simulink model "flightSimulation"  (R2018a)
settings: Solver=FixedStepAuto  StartTime=0  StopTime=end_time  FixedStep=0.005  RelTol=1e-3  EnableMultiTasking=on
values from neighbouring files (symbols this model uses):
  initPosLLA = [37.6287386167 -122.393391133 100]    [cmdh.mat]    (also in cmdyaw.mat)
  mass = 1.53    [cmdh.mat]    (also in cmdyaw.mat)
  Ts = 0.01    [cmdh.mat]    (also in cmdyaw.mat)
undefined symbols (not defined in the file or in its folder): B, Earth, ft, m, p_limits, s, sigbuilder_block, sw_turb, umax, umin, Vehicle, WGS84
libraries: simulink x23, aerolibactuator x15, dspswit3 x12, dspsrcs4 x10, dsparch4 x7, aerolibconvert2 x4, aerolibanimutils x2, qcatlib x2, aerolibfltsims x2, aerolibutil x2, shared6dof x1, aerolibtransform2 x1
(part 4 of 4)

== matlab function flightSimulation/Subsystem/ADRC_allocator1/MATLAB Function ==
  data: x1_d input; u_r output; x2_d input; x1 input; x2 input
function u_r = NLSEF_yaw(x1_d,x2_d,x1,x2)
e1=x1_d-x1;
if e1<-pi
    a1=e1+2*pi;
elseif e1>=pi
    a1=e1-2*pi;
else   
    a1=e1;
end
e2=x2_d-x2;
% kp=0.5;kd=0.5;% 限11
% kp=1;kd=1; % 限20
kp=0.5;kd=0.5;% 噪声
alfa1=0.75;alfa2=1.5;
delta=0.1;
u_r = kp*fal(a1,alfa1,delta)+kd*fal(e2,alfa2,delta); 
% kp=0.5;kd=0.5;
% u_r = kp*a1+kd*e2;   % 控制输出
end

== matlab function flightSimulation/Subsystem/ADRC_allocator1/MATLAB Function2 ==
  data: x1_d input; u_q output; x2_d input; x1 input; x2 input
function u_q = NLSEF_pitch(x1_d,x2_d,x1,x2)
e1=x1_d-x1;
e2=x2_d-x2;
% kp=1;kd=1.5;% 限11
% kp=1.5;kd=2;% 限20
kp=1;kd=1;% 噪声
alfa1=0.75;alfa2=1.5;
delta=0.1;
u_q = kp*fal(e1,alfa1,delta)+kd*fal(e2,alfa2,delta);   % 控制输出
% kp=0.4;kd=0.4;
% u_q = kp*e1+kd*e2;   % 控制输出
end

== matlab function flightSimulation/Subsystem/ADRC_allocator1/MATLAB Function3 ==
  data: x1_d input; u_p output; x2_d input; x1 input; x2 input
function u_p = NLSEF_roll(x1_d,x2_d,x1,x2)
e1=x1_d-x1;
e2=x2_d-x2;
% kp=1;kd=1.5;% 限11
% kp=1.5;kd=2;% 限20
kp=1;kd=1;% 噪声
alfa1=0.75;alfa2=1.5;
delta=0.1;
u_p = kp*fal(e1,alfa1,delta)+kd*fal(e2,alfa2,delta);   % 控制输出
% kp=0.4;kd=0.4;
% u_p = kp*e1+kd*e2;   % 控制输出
end

== matlab function flightSimulation/Subsystem/PID_allocator1/舵机偏角输入eso/MATLAB Function2 ==
  data: u input; y output
function y = fcn(u)
U1=u(1);
U2=u(2);
U3=u(3);
A=0.3491;

D=[-1  0  1;
    0 -1  1;
    1  0  1;
    0  1  1];
% D
D_=1*[-0.5000         0              0.5000         0;
         0           -0.5000         0              0.5000;
       0.2500         0.2500         0.2500         0.2500];
% pinv(D)
kc1=2.7;% 2.8
kc2=3.2;% 3.3
l_1=0.17078793;
l_2=0.06647954;
K=1*[-kc1*l_1    0        kc1*l_1     0;
      0      -kc1*l_1     0        kc1*l_1;
      kc2*l_2   kc2*l_2    kc2*l_2    kc2*l_2];
K_=pinv(K);
I_x=0.025483;
I_y=0.025504;
I_z=0.00562;
I=[I_x 0 0;0 I_y 0;0 0 I_z];
a=A-abs(U1);
b=A-abs(U2);
D_s=[-1  0 (2*a)/(a+b);
      0 -1  (2*b)/(a+b);
      1  0  (2*a)/(a+b);
      0  1 (2*b)/(a+b)];
    D=[-1  0  1;
      0 -1  1;
      1  0  1;
      0  1  1];
y=zeros(3,1);
y=I\(K*D)*([U1;U2;U3]);% K*D=K*D_s
% I\(K*D)*([U1;U2;U3])=扰动角加速度

== matlab function flightSimulation/Subsystem/ADRC_allocator1/Subsystem2/control allocation/inv/inv ==
  data: u input; y output
function y = fcn(u)
U = [u(1);u(2);u(3)];
y=zeros(4,1);
% M=crossover_point([0;0;0],e);
% if (norm(e)>norm(M))
%     U=M;
% else
%     U=e;
% end 
% B=[-0.5   0       0.5   0;
%     0  -0.5    0       0.5;
%     0.25   0.25   0.25   0.25];
kc1=3.157;% 2.8
kc2=3.157;% 3.3
l_1=0.17078793;
l_2=0.06647954;
B=1*[-kc1*l_1    0        kc1*l_1     0;
      0      -kc1*l_1     0        kc1*l_1;
      kc2*l_2   kc2*l_2    kc2*l_2    kc2*l_2];  
% u(1)=Constrain(u(1),umin(1),umax(1));
% u(2)=Constrain(u(2),umin(2),umax(2));
% u(3)=Constrain(u(3),umin(3),umax(3));
% u(4)=Constrain(u(4),umin(4),umax(4));
c=pinv(B)*U;
y=[c(1);c(2);c(3);c(4)];

== matlab function flightSimulation/Subsystem/PID/MATLAB Function ==
  data: u input; y output
function y = Eulerrate2pqr(u)
Roll=u(4);
Pitch=u(5);
Q=[1    sin(Roll)*tan(Pitch)    cos(Roll)*tan(Pitch);
   0        cos(Roll)               -sin(Roll);
   0    sin(Roll)*sec(Pitch)    cos(Roll)*sec(Pitch)];
y = Q\[u(1);u(2);u(3)];

== matlab function flightSimulation/Subsystem/PID/MATLAB Function1 ==
  data: u input; y output
function y = Yawcontrol(u)
if u<-pi
    a=u+2*pi;
elseif u>=pi
    a=u-2*pi;
else   
    a=u;
end
y = a;

== matlab function flightSimulation/Subsystem/ADRC_allocator/MATLAB Function ==
  data: x1_d input; u_r output; x2_d input; x1 input; x2 input
function u_r = NLSEF_yaw(x1_d,x2_d,x1,x2)
e1=x1_d-x1;
if e1<-pi
    a1=e1+2*pi;
elseif e1>=pi
    a1=e1-2*pi;
else   
    a1=e1;
end
e2=x2_d-x2;
kp=0.5;kd=0.5;
% kp=1;kd=1;
alfa1=0.75;alfa2=1.5;
delta=0.1;
u_r = kp*fal(a1,alfa1,delta)+kd*fal(e2,alfa2,delta); 
% kp=0.5;kd=0.5;
% u_r = kp*a1+kd*e2;   % 控制输出
end

== matlab function flightSimulation/Subsystem/ADRC_allocator/MATLAB Function2 ==
  data: x1_d input; u_q output; x2_d input; x1 input; x2 input
function u_q = NLSEF_pitch(x1_d,x2_d,x1,x2)
e1=x1_d-x1;
e2=x2_d-x2;
kp=1;kd=1.5;
% kp=1.5;kd=2;
alfa1=0.75;alfa2=1.5;
delta=0.1;
u_q = kp*fal(e1,alfa1,delta)+kd*fal(e2,alfa2,delta);   % 控制输出
% kp=0.4;kd=0.4;
% u_q = kp*e1+kd*e2;   % 控制输出
end

== matlab function flightSimulation/Subsystem/ADRC_allocator/MATLAB Function3 ==
  data: x1_d input; u_p output; x2_d input; x1 input; x2 input
function u_p = NLSEF_roll(x1_d,x2_d,x1,x2)
e1=x1_d-x1;
e2=x2_d-x2;
kp=1;kd=1.5;
% kp=1.5;kd=2;
alfa1=0.75;alfa2=1.5;
delta=0.1;
u_p = kp*fal(e1,alfa1,delta)+kd*fal(e2,alfa2,delta);   % 控制输出
% kp=0.4;kd=0.4;
% u_p = kp*e1+kd*e2;   % 控制输出
end

== matlab function flightSimulation/Subsystem/ADRC_allocator/Subsystem2/inv ==
  data: u input; y output
function y = fcn(u)
U = [u(1);u(2);u(3)];
y=zeros(4,1);
% M=crossover_point([0;0;0],e);
% if (norm(e)>norm(M))
%     U=M;
% else
%     U=e;
% end 
% B=[-0.5   0       0.5   0;
%     0  -0.5    0       0.5;
%     0.25   0.25   0.25   0.25];
kc1=3.157;% 2.8
kc2=3.157;% 3.3
l_1=0.17078793;
l_2=0.06647954;
B=1*[-kc1*l_1    0        kc1*l_1     0;
      0      -kc1*l_1     0        kc1*l_1;
      kc2*l_2   kc2*l_2    kc2*l_2    kc2*l_2];  
% u(1)=Constrain(u(1),umin(1),umax(1));
% u(2)=Constrain(u(2),umin(2),umax(2));
% u(3)=Constrain(u(3),umin(3),umax(3));
% u(4)=Constrain(u(4),umin(4),umax(4));
c=pinv(B)*U;
y=[c(1);c(2);c(3);c(4)];
